simulink model "m_modelcov02_harness"  (Simulink 8.0)
settings: Solver=FixedStepDiscrete  StartTime=0.0  StopTime=1  FixedStep=0.1  RelTol=1e-3
undefined symbols (not defined in the file or in its folder): sigbuilder_block
libraries: simulink x1
settings Model: SldvGeneratedHarnessModel=TestUnitModel=m_modelcov02|  Creator=The MathWorks Inc.  LastModifiedBy=itoy  RecordCoverage=on  CovMetricSettings=dcmoe  CovHTMLOptions=-aTS=1 -bRG=1 -bTC=0 -hTR=0 -nFC=0 -scm=1 -bcm=1  covSaveCumulativeToWorkspaceVar=off  CovSaveSingleToWorkspaceVar=off  CovModelRefEnable=off  CovExternalEMLEnable=on
settings DataIOCC: LimitDataPoints=off  SaveFormat=StructureWithTime  SignalLoggingSaveFormat=ModelDataLogs  SaveOutput=off  SaveTime=off
settings OptimizationCC: ConditionallyExecuteInputs=off  InlineParams=on  InlineInvariantSignals=on  InitFltsAndDblsToZero=on  EfficientMapNaN2IntZero=off
settings DebuggingCC: SaveWithParameterizedLinksMsg=none  SignalResolutionControl=TryResolveAllWithWarning  InheritedTsInSrcMsg=none  FcnCallInpInsideContextMsg=UseLocalSettings  StrictBusMsg=Warning
settings GRTTargetCC: TargetFcnLib=ansi_tfl_tmw.mat  CombineOutputUpdateFcns=off  GRTInterface=on
settings ConfigComp: Description=Design Verifier Custom Configuration Component  DVMaxProcessTime=60  DVMakeOutputFilesUnique=off  DVParameters=on  DVModelCoverageObjectives=MCDC  DVMaxTestCaseSteps=500  DVTestSuiteOptimization=CombinedObjectives  DVAssertions=EnableAll  DVProofAssumptions=EnableAll  DVProvingStrategy=FindViolation

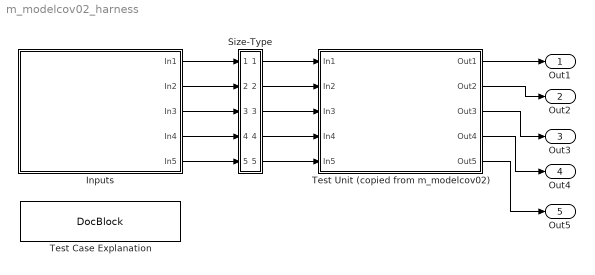
== system m_modelcov02_harness ==
  Inputs : Subsystem  Tag=STV Subsys  LoadFcn=sigbuilder_block('load',[49.5 50.25 519.75 399.75 ]);  StartFcn=sigbuilder_block('start');  StopFcn=sigbuilder_block('stop');  ClipboardFcn=sigbuilder_block('clipboard');  mask(Sigbuilder block){}
      mask init:
      | if ~strcmp(get_param(bdroot(gcb),'SimulationStatus'),'stopped'),tuvar = sigbuilder_block('maskInit'); end
      settings: CopyFcn=sigbuilder_block('copy');  DeleteFcn=sigbuilder_block('delete');  ModelCloseFcn=sigbuilder_block('modelClose');  PreSaveFcn=sigbuilder_block('preSave');  PauseFcn=sigbuilder_block('pause');  ContinueFcn=sigbuilder_block('continue');  NameChangeFcn=sigbuilder_block('namechange');  OpenFcn=sigbuilder_block('open');  CloseFcn=sigbuilder_block('close');
      mask Display: plot(0, 0, 100, 100,[2, 2, 32, 32, 2], [68, 8, 8, 68, 68],[32, 2], [38, 38], [32, 19, 2],[53, 60, 44], [32, 17, 17, 2],[16, 16, 31, 31]);txt = getActiveGroup(gcbh);text(2, 100, txt,'verticalAlignment', 'top');
  Size-Type : Subsystem
  Test Case Explanation : simulink/Model-Wide Utilities/DocBlock  DocumentType=Text
  Test Unit (copied from m_modelcov02) : Subsystem
  Out1 : Outport
  Out2 : Outport  Port=2
  Out3 : Outport  Port=3
  Out4 : Outport  Port=4
  Out5 : Outport  Port=5
  wires:
  Inputs/1(In1) -> Size-Type/1(In1)
  Size-Type/1(Out1) -> Test Unit (copied from m_modelcov02)/1(In1)
  Inputs/2(In2) -> Size-Type/2(In2)
  Size-Type/2(Out2) -> Test Unit (copied from m_modelcov02)/2(In2)
  Inputs/3(In3) -> Size-Type/3(In3)
  Size-Type/3(Out3) -> Test Unit (copied from m_modelcov02)/3(In3)
  Inputs/4(In4) -> Size-Type/4(In4)
  Size-Type/4(Out4) -> Test Unit (copied from m_modelcov02)/4(In4)
  Inputs/5(In5) -> Size-Type/5(In5)
  Size-Type/5(Out5) -> Test Unit (copied from m_modelcov02)/5(In5)
  Test Unit (copied from m_modelcov02)/1(Out1) -> Out1/1
  Test Unit (copied from m_modelcov02)/2(Out2) -> Out2/1
  Test Unit (copied from m_modelcov02)/3(Out3) -> Out3/1
  Test Unit (copied from m_modelcov02)/4(Out4) -> Out4/1
  Test Unit (copied from m_modelcov02)/5(Out5) -> Out5/1

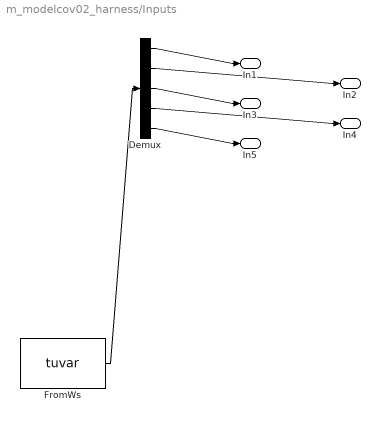
== system m_modelcov02_harness/Inputs ==
  Demux : Demux  Tag=STV Demux  Outputs=5
  FromWs : FromWorkspace  Tag=STV FromWs  VariableName=tuvar  SampleTime=0  SigBuilderData=DataTag0  VnvData=DataTag1
      SigBuilderData=|
      | dataSet.timeRange = [0 0.1]
      | dataSet.name = 'Test Case 1'
      | sbobj.Name = 'Signal Builder'
      | sbobj.Groups.Name = 'Test Case 1'
      | sbobj.Groups.Signals(1).Name = 'In1'
      | sbobj.Groups.Signals(1).XData = [0 0.1]
      | sbobj.Groups.Signals(1).YData = [0 0]
      | sbobj.Groups.Signals(2).Name = 'In2'
      | sbobj.Groups.Signals(2).XData = [0 0.1]
      | sbobj.Groups.Signals(2).YData = [0 0]
      | sbobj.Groups.Signals(3).Name = 'In3'
      | sbobj.Groups.Signals(3).XData = [0 0.1]
      | sbobj.Groups.Signals(3).YData = [0 0]
      | sbobj.Groups.Signals(4).Name = 'In4'
      | sbobj.Groups.Signals(4).XData = [0 0.1]
      | sbobj.Groups.Signals(4).YData = [0 0]
      | sbobj.Groups.Signals(5).Name = 'In5'
      | sbobj.Groups.Signals(5).XData = [0 0.1]
      | sbobj.Groups.Signals(5).YData = [0 0]
      | sbobj.Groups.TimeRange = [0 0.1]
  In1 : Outport  Tag=STV Outport
  In2 : Outport  Tag=STV Outport  Port=2
  In3 : Outport  Tag=STV Outport  Port=3
  In4 : Outport  Tag=STV Outport  Port=4
  In5 : Outport  Tag=STV Outport  Port=5
  wires:
  FromWs/1 -> Demux/1
  Demux/1 -> In1/1
  Demux/2 -> In2/1
  Demux/3 -> In3/1
  Demux/4 -> In4/1
  Demux/5 -> In5/1

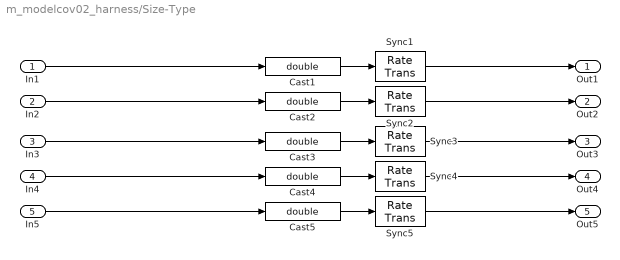
== system m_modelcov02_harness/Size-Type ==
  In1 : Inport
  In2 : Inport  Port=2
  In3 : Inport  Port=3
  In4 : Inport  Port=4
  In5 : Inport  Port=5
  Cast{1..5} (5 alike) : DataTypeConversion  OutDataTypeStr=double  SaturateOnIntegerOverflow=on  RndMeth=Zero
  Sync{1..5} (5 alike) : RateTransition  OutPortSampleTime=[0.10000000000000001,0]
  Out1 : Outport
  Out2 : Outport  Port=2
  Out3 : Outport  Port=3
  Out4 : Outport  Port=4
  Out5 : Outport  Port=5
  wires:
  In1/1 -> Cast1/1
  Cast1/1 -> Sync1/1
  Sync1/1 -> Out1/1
  In2/1 -> Cast2/1
  Cast2/1 -> Sync2/1
  Sync2/1 -> Out2/1
  In3/1 -> Cast3/1
  Cast3/1 -> Sync3/1
  Sync3/1 -> Out3/1
  In4/1 -> Cast4/1
  Cast4/1 -> Sync4/1
  Sync4/1 -> Out4/1
  In5/1 -> Cast5/1
  Cast5/1 -> Sync5/1
  Sync5/1 -> Out5/1

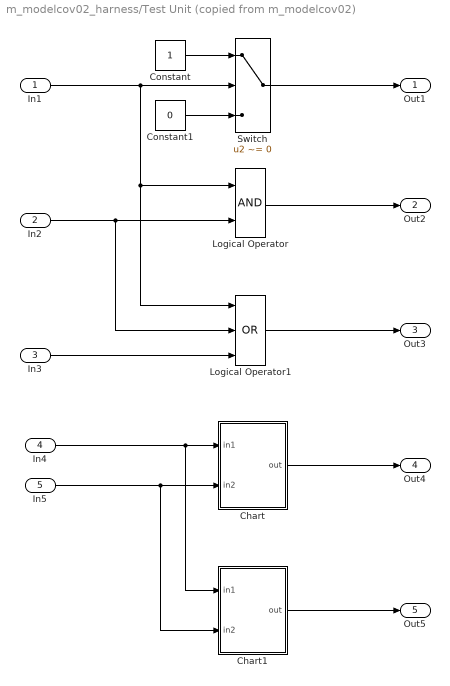
== system m_modelcov02_harness/Test Unit (copied from m_modelcov02) ==
  In1 : Inport
  In2 : Inport  Port=2
  In3 : Inport  Port=3
  In4 : Inport  Port=4
  In5 : Inport  Port=5
  Chart : Stateflow chart  TreatAsAtomicUnit=on
  Chart1 : Stateflow chart  TreatAsAtomicUnit=on
  Constant : Constant
  Constant1 : Constant  Value=0
  Logical Operator : Logic  AllPortsSameDT=off  OutDataTypeStr=boolean
  Logical Operator1 : Logic  Operator=OR  Inputs=3  AllPortsSameDT=off  OutDataTypeStr=boolean
  Switch : Switch  Criteria=u2 ~= 0
  Out1 : Outport
  Out2 : Outport  Port=2
  Out3 : Outport  Port=3
  Out4 : Outport  Port=4
  Out5 : Outport  Port=5
  wires:
  Chart1/1(out) -> Out5/1
  Chart/1(out) -> Out4/1
  In5/1 -> Chart1/2(in2), Chart/2(in2)
  In4/1 -> Chart1/1(in1), Chart/1(in1)
  Logical Operator1/1 -> Out3/1
  Logical Operator/1 -> Out2/1
  In3/1 -> Logical Operator1/3
  In2/1 -> Logical Operator1/2, Logical Operator/2
  Switch/1 -> Out1/1
  Constant1/1 -> Switch/3
  In1/1 -> Logical Operator/1, Logical Operator1/1, Switch/2
  Constant/1 -> Switch/1

== stateflow chart Test Unit (copied from m_modelcov02)/Chart ==
  state P/
    state A/
      out = 1;
    state B/
      out = 0;
    (default) -> A
    A -> B : [ in1 == 0 ]
    B -> A : [ in1 ~= 0 ]
  state C/
    out = 2;
  (default) -> P
  C -> A : [in2 ~= 1]
  P -> C : [in2 == 1]
  data: in1 input double; in2 input double; out output uint8

== stateflow chart Test Unit (copied from m_modelcov02)/Chart1 ==
  (default) -> (junction 22)
  (junction 22) -> (junction 21) [order 1] : [ in1 == 1 && in2 == 0 ]
  (junction 21) -> (junction 24) : {
      | out = 0;
      | }
  (junction 22) -> (junction 23) [order 2] : {
      | out = 1;
      | }
  data: in1 input double; in2 input double; out output uint8
